simulink model "i_128w_2k_10_r310"  (Simulink 7.0)
settings: Solver=ode45  StartTime=0.0  StopTime=100000  RelTol=1e-3
undefined symbols (not defined in the file or in its folder): iBOB
libraries: xbsIndex_r4 x626, xps_library x14, xbsReplacements_r4 x12, casper_library x6, casper_library_sources x4, simulink x1
(part 1 of 6)
settings Model: Creator=dsp  LastModifiedBy=mdexter

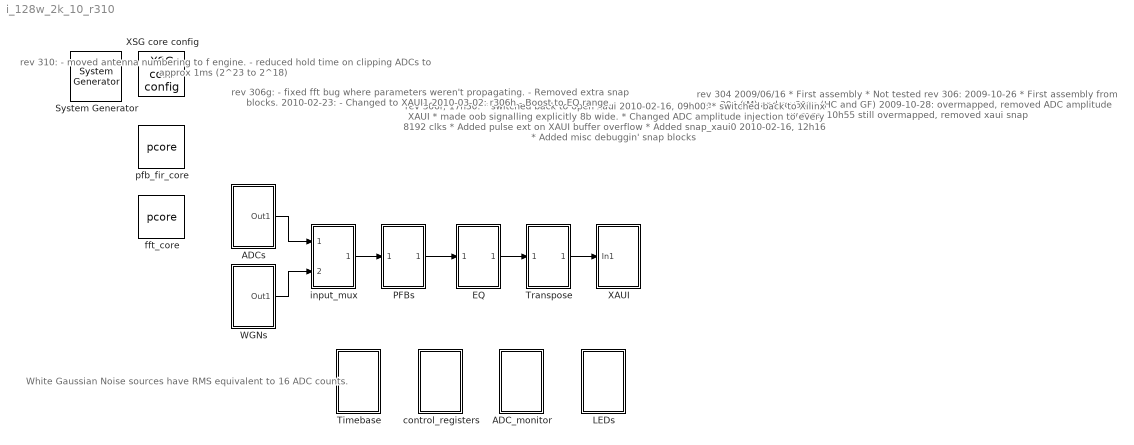
== system i_128w_2k_10_r310 ==
  note: rev 304 2009/06/16
      | * First assembly
      | * Not tested
      |
      | rev 306: 2009-10-26
      | * First assembly from rev 304 (JM) and rev305c (HC and GF)
      |
      | 2009-10-28: overmapped, removed ADC amplitude sw regs.
      | 10h55 still overmapped, removed xaui snap
  note: rev 306f, 17h30:
      |   * switched back to open xaui
      | 2010-02-16, 09h00:
      |   * switched back to Xilinx XAUI
      |   * made oob signalling explicitly 8b wide.
      |   * Changed ADC amplitude injection to every 8192 clks
      |   * Added pulse ext on XAUI buffer overflow
      |   * Added snap_xaui0
      | 2010-02-16, 12h16
      |   * Added misc debuggin' snap blocks
  note: rev 306g:
      |  - fixed fft bug where parameters
      |     weren't propagating.
      |   - Removed extra snap blocks.
      |
      | 2010-02-23:
      |   - Changed to XAUI1
      |
      | 2010-03-02: r306h
      |   - Boost to EQ range.
  note: rev 310:
      |  - moved antenna numbering to
      |    f engine.
      |  - reduced hold time on clipping
      |    ADCs to approx 1ms (2^23 to 2^18)
  note: White Gaussian Noise
      | sources have RMS
      | equivalent to 16 ADC
      | counts.
  " System Generator" : xbsIndex_r4/ System Generator  Tag=genX  SystemSampleTime=-1  xilinxfamily=virtex2p  part=xc2vp50  speed=-7  package=ff1152  synthesis_tool=XST  clock_wrapper=Clock Enables  directory=./i_128w_2k_10_r310/sysgen  testbench=off  simulink_period=1  sysclk_period=5  dcm_input_clock_period=100  incr_netlist=off  trim_vbits=Everywhere in SubSystem  dbl_ovrd=According to Block Masks  core_generation=According to Block Masks  run_coregen=off  deprecated_control=off  eval_field=0  block_type=sysgen
      settings: block_version=10.1.3
  ADC_monitor : Subsystem
  ADCs : Subsystem
  EQ : Subsystem
  LEDs : Subsystem
  PFBs : Subsystem
  Timebase : Subsystem
  Transpose : Subsystem
  WGNs : Subsystem
  XAUI : Subsystem
  XSG core config : xps_library/XSG core config  Tag=xps:xsg  SystemSampleTime=-1  hw_sys=iBOB  ibob_linux=off  clk_src=adc0_clk  iBOB_clk_src=adc0_clk  BEE2_ctrl_clk_src=sys_clk  BEE2_usr_clk_src=sys_clk  ROACH_clk_src=arb_clk  CORR_clk_src=sys_clk  gpio_clk_io_group=iBOB:sma  gpio_clk_bit_index=0  clk_rate=200  sample_period=1  synthesis_tool=XST  mpc_type=powerpc405
  control_registers : Subsystem
  fft_core : xps_library/pcore  Tag=xps:pcore  SystemSampleTime=-1  pcore_path=fft_core/fft_core.ngc
  input_mux : Subsystem
  pfb_fir_core : xps_library/pcore  Tag=xps:pcore  SystemSampleTime=-1  pcore_path=pfb_fir_core/pfb_fir_core.ngc
  wires:
  ADCs/1(Out1) -> input_mux/1(In1)
  WGNs/1(Out1) -> input_mux/2(In2)
  input_mux/1(Out1) -> PFBs/1(In1)
  PFBs/1(Out1) -> EQ/1(In1)
  EQ/1(Out1) -> Transpose/1(In1)
  Transpose/1(Out1) -> XAUI/1(In1)

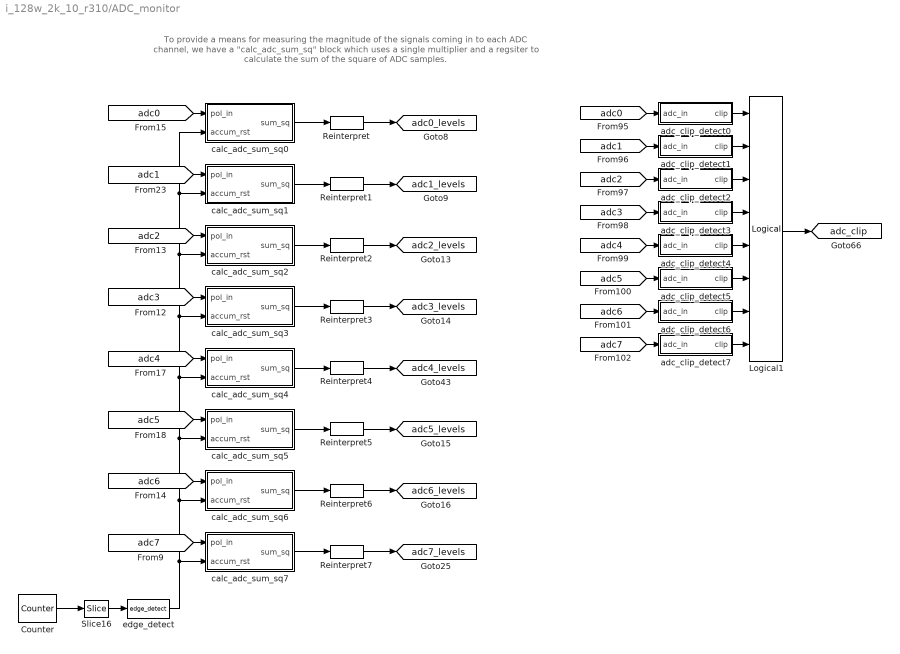
== system i_128w_2k_10_r310/ADC_monitor ==
  note: To provide a means for measuring the magnitude of the signals
      | coming in to each ADC channel, we have a "calc_adc_sum_sq"
      | block which uses a single multiplier and a regsiter to calculate
      | the sum of the square of ADC samples.
  Counter : xbsIndex_r4/Counter  cnt_type=Free Running  cnt_to=Inf  operation=Up  start_count=0  cnt_by_val=1  arith_type=Unsigned  n_bits=16  bin_pt=0  load_pin=off  rst=off  en=off  explicit_period=off  period=1  dbl_ovrd=off  use_behavioral_HDL=off  use_rpm=on  implementation=Fabric  block_type=counter
      settings: xl_area=[0, 0, 0, 0, 0, 0, 0]
  Logical1 : xbsIndex_r4/Logical  logical_function=OR  inputs=8  en=off  latency=1  precision=Full  arith_type=Unsigned  n_bits=8  bin_pt=2  align_bp=on  dbl_ovrd=off  block_type=logical
      settings: xl_area=[0, 0, 0, 0, 0, 0, 0]
  Reinterpret{,1..7} (8 alike) : xbsIndex_r4/Reinterpret  force_arith_type=on  arith_type=Unsigned  force_bin_pt=on  bin_pt=0  block_type=reinterpret
      settings: infoedit="Changes signal type without altering the binary representation.   You can changed the signal between signed and unsigned, and relocate the binary point.<P><P>Hardware notes: In hardware this block costs nothing.<P><P>Example:  Suppose the input is 6 bits wide, signed, with 2 fractional bits, and the output is forced to unsigned with 0 fractional bits.  Then an input of -2.0 (1110.00 in binary 2's complement) becomes an output of 56 (111000 in binary)."  block_version=10.1.3
  Slice16 : xbsIndex_r4/Slice  nbits=1  boolean_output=on  mode=Upper Bit Location + Width  bit1=0  base1=MSB of Input  bit0=19  base0=LSB of Input  dbl_ovrd=off  block_type=slice
      settings: infoedit="Extracts a given range of bits from each input sample and presents it at the output.  The output type is ordinarily unsigned with binary point at zero, but can be Boolean when the slice is one bit wide.<P><P>Hardware notes: In hardware this block costs nothing."  block_version=10.1.3
  adc_clip_detect0 : Subsystem  mask{n_bits=8}
      mask prompts: n_bits "Number of ADC bits"
  adc_clip_detect1 : Subsystem  mask{n_bits=8}
      mask prompts: n_bits "Number of ADC bits"
  adc_clip_detect2 : Subsystem  mask{n_bits=8}
      mask prompts: n_bits "Number of ADC bits"
  adc_clip_detect3 : Subsystem  mask{n_bits=8}
      mask prompts: n_bits "Number of ADC bits"
  adc_clip_detect4 : Subsystem  mask{n_bits=8}
      mask prompts: n_bits "Number of ADC bits"
  adc_clip_detect5 : Subsystem  mask{n_bits=8}
      mask prompts: n_bits "Number of ADC bits"
  adc_clip_detect6 : Subsystem  mask{n_bits=8}
      mask prompts: n_bits "Number of ADC bits"
  adc_clip_detect7 : Subsystem  mask{n_bits=8}
      mask prompts: n_bits "Number of ADC bits"
  calc_adc_sum_sq0 : Subsystem
  calc_adc_sum_sq1 : Subsystem
  calc_adc_sum_sq2 : Subsystem
  calc_adc_sum_sq3 : Subsystem
  calc_adc_sum_sq4 : Subsystem
  calc_adc_sum_sq5 : Subsystem
  calc_adc_sum_sq6 : Subsystem
  calc_adc_sum_sq7 : Subsystem
  edge_detect : casper_library/Misc/edge_detect  SystemSampleTime=-1  edge=Rising  polarity=Active High  x_in=[0 0.08 0.08 0.16 0.16 0.24 0.24 0.32 0.32 0.4]  y_in="[-1 -1  1  1  1  1  1  1  1  1]"  x_out=[0.6 0.68 0.68 0.76 0.76 0.84 0.84 0.92 0.92 1]  y_out="[-1 -1  1  1 -1 -1 -1 -1 -1 -1]"
      settings: AttributesFormatString=|
      | rising edges
      | active high
  tag scope: adc0_levels=global, adc1_levels=global, adc2_levels=global, adc3_levels=global, adc4_levels=global, adc5_levels=global, adc6_levels=global, adc7_levels=global, adc_clip=global
  wires:
  [adc0] -> calc_adc_sum_sq0/1(pol_in)
  calc_adc_sum_sq1/1(sum_sq) -> Reinterpret1/1
  calc_adc_sum_sq2/1(sum_sq) -> Reinterpret2/1
  calc_adc_sum_sq3/1(sum_sq) -> Reinterpret3/1
  edge_detect/1 -> calc_adc_sum_sq0/2(accum_rst), calc_adc_sum_sq1/2(accum_rst), calc_adc_sum_sq2/2(accum_rst), calc_adc_sum_sq3/2(accum_rst), calc_adc_sum_sq4/2(accum_rst), calc_adc_sum_sq5/2(accum_rst), calc_adc_sum_sq6/2(accum_rst), calc_adc_sum_sq7/2(accum_rst)
  [adc1] -> calc_adc_sum_sq1/1(pol_in)
  [adc2] -> calc_adc_sum_sq2/1(pol_in)
  [adc3] -> calc_adc_sum_sq3/1(pol_in)
  Counter/1 -> Slice16/1
  Slice16/1 -> edge_detect/1
  calc_adc_sum_sq4/1(sum_sq) -> Reinterpret4/1
  [adc4] -> calc_adc_sum_sq4/1(pol_in)
  calc_adc_sum_sq5/1(sum_sq) -> Reinterpret5/1
  calc_adc_sum_sq6/1(sum_sq) -> Reinterpret6/1
  calc_adc_sum_sq7/1(sum_sq) -> Reinterpret7/1
  [adc5] -> calc_adc_sum_sq5/1(pol_in)
  [adc6] -> calc_adc_sum_sq6/1(pol_in)
  [adc7] -> calc_adc_sum_sq7/1(pol_in)
  Reinterpret/1 -> [adc0_levels]
  Reinterpret1/1 -> [adc1_levels]
  Reinterpret2/1 -> [adc2_levels]
  Reinterpret3/1 -> [adc3_levels]
  Reinterpret4/1 -> [adc4_levels]
  Reinterpret5/1 -> [adc5_levels]
  Reinterpret6/1 -> [adc6_levels]
  Reinterpret7/1 -> [adc7_levels]
  calc_adc_sum_sq0/1(sum_sq) -> Reinterpret/1
  [adc0] -> adc_clip_detect0/1(adc_in)
  [adc1] -> adc_clip_detect1/1(adc_in)
  [adc2] -> adc_clip_detect2/1(adc_in)
  [adc3] -> adc_clip_detect3/1(adc_in)
  [adc4] -> adc_clip_detect4/1(adc_in)
  [adc5] -> adc_clip_detect5/1(adc_in)
  [adc6] -> adc_clip_detect6/1(adc_in)
  [adc7] -> adc_clip_detect7/1(adc_in)
  adc_clip_detect0/1(clip) -> Logical1/1
  adc_clip_detect1/1(clip) -> Logical1/2
  adc_clip_detect2/1(clip) -> Logical1/3
  adc_clip_detect3/1(clip) -> Logical1/4
  adc_clip_detect4/1(clip) -> Logical1/5
  adc_clip_detect5/1(clip) -> Logical1/6
  adc_clip_detect6/1(clip) -> Logical1/7
  adc_clip_detect7/1(clip) -> Logical1/8
  Logical1/1 -> [adc_clip]

== system i_128w_2k_10_r310/ADCs ==
  Band-Limited White Noise : simulink/Sources/Band-Limited White Noise  SystemSampleTime=-1  Cov=[0.1]  Ts=0.1  seed=[23341]
  Constant : Constant  Value=0
  Constant1 : Constant  OutDataType=sfix(16)  OutScaling=2^0
  Constant2 : Constant  Value=0
  Mux : Mux  Inputs=2
  Pulse Generator : DiscretePulseGenerator  Period=2^27
  Terminator11 : Terminator
  Terminator12 : Terminator
  quadc0 : xps_library/quadc  Tag=xps:quadc  SystemSampleTime=-1  adc_brd=0  adc_clk_rate=200
  quadc1 : xps_library/quadc  Tag=xps:quadc  SystemSampleTime=-1  adc_brd=1  adc_clk_rate=200
  Out1 : Outport  OutDataType=sfix(16)  OutScaling=2^0
  tag scope: adc0=global, adc1=global, adc2=global, adc3=global, adc4=global, adc5=global, adc6=global, adc7=global, sync_adc0=global, sync_adc1=global
  wires:
  quadc0/1 -> [adc0]
  quadc0/2 -> [adc1]
  quadc0/3 -> [adc2]
  quadc0/4 -> [adc3]
  quadc0/6 -> [sync_adc0]
  quadc1/1 -> [adc4]
  quadc1/2 -> [adc5]
  quadc1/3 -> [adc6]
  quadc1/4 -> [adc7]
  quadc1/6 -> [sync_adc1]
  Band-Limited White Noise/1 -> quadc1/4, quadc1/3, quadc1/2, quadc1/1, quadc0/4, quadc0/3, quadc0/2, quadc0/1
  Pulse Generator/1 -> quadc0/6, quadc1/6
  Constant1/1 -> quadc0/5, quadc1/5
  quadc0/5 -> Terminator11/1
  quadc1/5 -> Terminator12/1
  Mux/1 -> Out1/1
  Constant/1 -> Mux/1
  Constant2/1 -> Mux/2

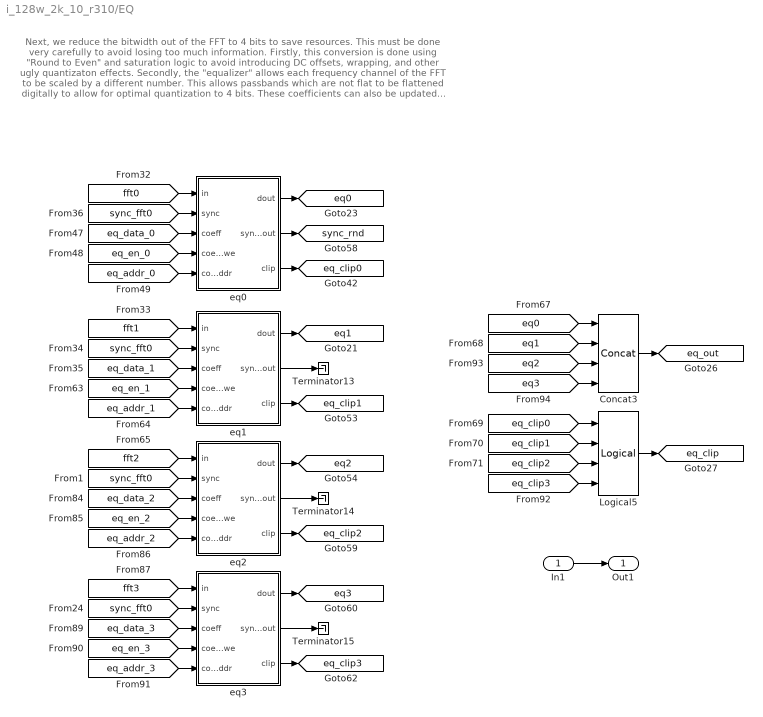
== system i_128w_2k_10_r310/EQ ==
  note: Next, we reduce the bitwidth out of the FFT to 4 bits to save resources.
      | This must be done very carefully to avoid losing too much information.
      | Firstly, this conversion is done using "Round to Even" and saturation
      | logic to avoid introducing DC offsets, wrapping, and other ugly quantizaton
      | effects.  Secondly, the "equalizer" allows each frequency channel of the
      | FFT to be scaled by a different number.  This allows passbands which are
      | not flat to be flattened digitally to allow for optimal quantization to 4 bits.
      | These coefficients can also be updated dynamically for gain control.
      | Coefficients can be dynamically written into the "equalizer" by
      | specifying the channel ("coeff_addr") and the value of the
      | coefficient ("coeff"), and then using "coeff_en" to write the
      | new coefficient into the equalization table.
  In1 : Inport  OutDataType=sfix(16)  OutScaling=2^0
  Concat3 : xbsIndex_r4/Concat  num_inputs=4  dbl_ovrd=off  block_type=concat
      settings: block_version=10.1.3
  Logical5 : xbsIndex_r4/Logical  logical_function=OR  inputs=4  en=off  latency=0  precision=Full  arith_type=Unsigned  n_bits=8  bin_pt=2  align_bp=on  dbl_ovrd=off  block_type=logical
      settings: xl_area=[0, 0, 0, 0, 0, 0, 0]
  Terminator13 : Terminator
  Terminator14 : Terminator
  Terminator15 : Terminator
  eq0 : Subsystem
  eq1 : Subsystem
  eq2 : Subsystem
  eq3 : Subsystem
  Out1 : Outport  OutDataType=sfix(16)  OutScaling=2^0
  tag scope: eq0=global, eq1=global, eq2=global, eq3=global, eq_clip0=global, eq_clip1=global, eq_clip2=global, eq_clip3=global, eq_clip=global, eq_out=global, sync_rnd=global
  wires:
  eq0/1(dout) -> [eq0]
  eq0/2(sync_out) -> [sync_rnd]
  [fft0] -> eq0/1(in)
  [eq_data_0] -> eq0/3(coeff)
  [eq_en_0] -> eq0/4(coeff_we)
  eq0/3(clip) -> [eq_clip0]
  Logical5/1 -> [eq_clip]
  Concat3/1 -> [eq_out]
  [eq_clip0] -> Logical5/1
  [eq_clip1] -> Logical5/2
  [sync_fft0] -> eq0/2(sync)
  [eq_addr_0] -> eq0/5(coeff_addr)
  [fft1] -> eq1/1(in)
  [sync_fft0] -> eq1/2(sync)
  [eq_data_1] -> eq1/3(coeff)
  [eq_en_1] -> eq1/4(coeff_we)
  [eq_addr_1] -> eq1/5(coeff_addr)
  [fft2] -> eq2/1(in)
  [sync_fft0] -> eq2/2(sync)
  [eq_data_2] -> eq2/3(coeff)
  [eq_en_2] -> eq2/4(coeff_we)
  [eq_addr_2] -> eq2/5(coeff_addr)
  [fft3] -> eq3/1(in)
  [sync_fft0] -> eq3/2(sync)
  [eq_data_3] -> eq3/3(coeff)
  [eq_en_3] -> eq3/4(coeff_we)
  [eq_addr_3] -> eq3/5(coeff_addr)
  eq1/1(dout) -> [eq1]
  eq1/2(sync_out) -> Terminator13/1
  eq1/3(clip) -> [eq_clip1]
  eq2/1(dout) -> [eq2]
  eq2/2(sync_out) -> Terminator14/1
  eq2/3(clip) -> [eq_clip2]
  eq3/1(dout) -> [eq3]
  eq3/2(sync_out) -> Terminator15/1
  eq3/3(clip) -> [eq_clip3]
  [eq_clip2] -> Logical5/3
  [eq_clip3] -> Logical5/4
  [eq0] -> Concat3/1
  [eq1] -> Concat3/2
  [eq2] -> Concat3/3
  [eq3] -> Concat3/4
  In1/1 -> Out1/1

== system i_128w_2k_10_r310/LEDs ==
  Terminator{1..5,27} (6 alike) : Terminator
  led1_arm : xps_library/gpio  Tag=xps:gpio  SystemSampleTime=-1  io_group=iBOB:led  io_dir=out  arith_type=Boolean  bitwidth=1  bin_pt=0  bit_index=1  sample_period=1  use_single_ended=off  use_ddr=off  reg_iob=on  reg_clk_phase=0  termination=None
      link override convert: arith_type=Boolean  n_bits=1  bin_pt=0
  led2_sync : xps_library/gpio  Tag=xps:gpio  SystemSampleTime=-1  io_group=iBOB:led  io_dir=out  arith_type=Boolean  bitwidth=1  bin_pt=0  bit_index=2  sample_period=1  use_single_ended=off  use_ddr=off  reg_iob=on  reg_clk_phase=0  termination=None
      link override convert: arith_type=Boolean  n_bits=1  bin_pt=0
  led4_eq_clip : xps_library/gpio  Tag=xps:gpio  SystemSampleTime=-1  io_group=iBOB:led  io_dir=out  arith_type=Boolean  bitwidth=1  bin_pt=0  bit_index=4  sample_period=1  use_single_ended=off  use_ddr=off  reg_iob=on  reg_clk_phase=0  termination=None
      link override convert: arith_type=Boolean  n_bits=1  bin_pt=0
  led5_adc_clip : xps_library/gpio  Tag=xps:gpio  SystemSampleTime=-1  io_group=iBOB:led  io_dir=out  arith_type=Boolean  bitwidth=1  bin_pt=0  bit_index=5  sample_period=1  use_single_ended=off  use_ddr=off  reg_iob=on  reg_clk_phase=0  termination=None
      link override convert: arith_type=Boolean  n_bits=1  bin_pt=0
  led6_link_dn : xps_library/gpio  Tag=xps:gpio  SystemSampleTime=-1  io_group=iBOB:led  io_dir=out  arith_type=Unsigned  bitwidth=1  bin_pt=0  bit_index=6  sample_period=1  use_single_ended=off  use_ddr=off  reg_iob=on  reg_clk_phase=0  termination=None
      link override convert: arith_type=Unsigned  n_bits=1  bin_pt=0
  led7_xaui_overlfow : xps_library/gpio  Tag=xps:gpio  SystemSampleTime=-1  io_group=iBOB:led  io_dir=out  arith_type=Unsigned  bitwidth=1  bin_pt=0  bit_index=7  sample_period=1  use_single_ended=off  use_ddr=off  reg_iob=on  reg_clk_phase=0  termination=None
      link override convert: arith_type=Unsigned  n_bits=1  bin_pt=0
  pulse_ext2 : Subsystem  mask{pulse_len=2^23}
      mask prompts: pulse_len "Length of Pulse"
      mask init:
      | bits = ceil(log2(pulse_len+1));
  pulse_ext3 : Subsystem  mask{pulse_len=2^18}
      mask prompts: pulse_len "Length of Pulse"
      mask init:
      | bits = ceil(log2(pulse_len+1));
  pulse_ext4 : Subsystem  mask{pulse_len=2^18}
      mask prompts: pulse_len "Length of Pulse"
      mask init:
      | bits = ceil(log2(pulse_len+1));
  wires:
  pulse_ext2/1(out) -> led2_sync/1
  [sync_gen] -> pulse_ext2/1(in)
  [armed] -> led1_arm/1
  [xaui_link_down] -> led6_link_dn/1
  pulse_ext4/1(out) -> led4_eq_clip/1
  [eq_clip] -> pulse_ext4/1(in)
  [xaui_buffer_overflow] -> led7_xaui_overlfow/1
  led1_arm/1 -> Terminator27/1
  led4_eq_clip/1 -> Terminator2/1
  led2_sync/1 -> Terminator3/1
  led6_link_dn/1 -> Terminator4/1
  led7_xaui_overlfow/1 -> Terminator5/1
  [adc_clip] -> pulse_ext3/1(in)
  pulse_ext3/1(out) -> led5_adc_clip/1
  led5_adc_clip/1 -> Terminator1/1

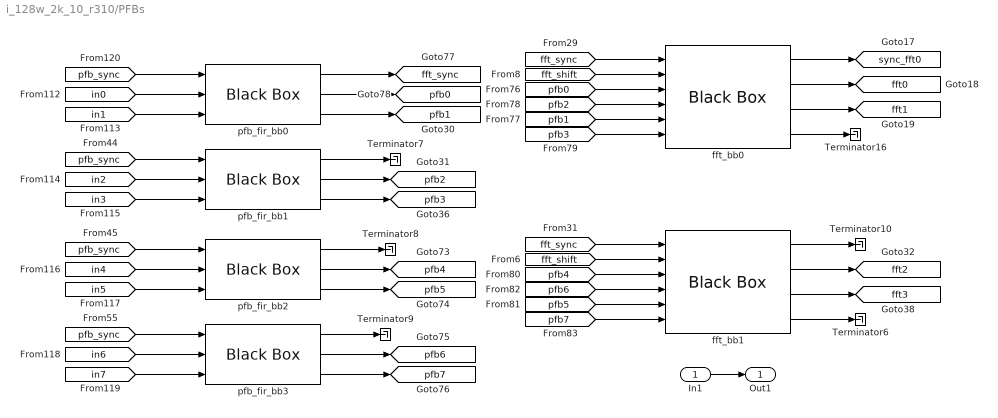
== system i_128w_2k_10_r310/PFBs ==
  In1 : Inport  OutDataType=sfix(16)  OutScaling=2^0
  Terminator{6..10,16} (6 alike) : Terminator
  fft_bb0 : xbsIndex_r4/Black Box  init_code=fft_core_config  sim_method=Inactive  block_type=blackbox2
      settings: infoedit="Incorporates black box HDL and simulation model into a System Generator design.<P><P>You must supply a Black Box with certain information about the HDL component you would like to bring into System Generator. This information is provided through a Matlab function.<P><P>When \"Simulation mode\" is set to \"Inactive\", you will typically want to provide a separate simulation model by using a Simulation Multiplexer.<P>When \"Simulation mode\" is set to \"External co-simulator\", you must include a ModelSim block in the design."  block_version=10.1.3
  fft_bb1 : xbsIndex_r4/Black Box  init_code=fft_core_config  sim_method=Inactive  block_type=blackbox2
      settings: infoedit="Incorporates black box HDL and simulation model into a System Generator design.<P><P>You must supply a Black Box with certain information about the HDL component you would like to bring into System Generator. This information is provided through a Matlab function.<P><P>When \"Simulation mode\" is set to \"Inactive\", you will typically want to provide a separate simulation model by using a Simulation Multiplexer.<P>When \"Simulation mode\" is set to \"External co-simulator\", you must include a ModelSim block in the design."  block_version=10.1.3
  pfb_fir_bb{0..3} (4 alike) : xbsIndex_r4/Black Box  init_code=pfb_fir_core_config  sim_method=Inactive  block_type=blackbox2
      settings: infoedit="Incorporates black box HDL and simulation model into a System Generator design.<P><P>You must supply a Black Box with certain information about the HDL component you would like to bring into System Generator. This information is provided through a Matlab function.<P><P>When \"Simulation mode\" is set to \"Inactive\", you will typically want to provide a separate simulation model by using a Simulation Multiplexer.<P>When \"Simulation mode\" is set to \"External co-simulator\", you must include a ModelSim block in the design."  block_version=10.1.3
  Out1 : Outport  OutDataType=sfix(16)  OutScaling=2^0
  tag scope: fft0=global, fft1=global, fft2=global, fft3=global, fft_sync=global, pfb0=global, pfb1=global, pfb2=global, pfb3=global, pfb4=global, pfb5=global, pfb6=global, pfb7=global, sync_fft0=global
  wires:
  [in0] -> pfb_fir_bb0/2
  [in1] -> pfb_fir_bb0/3
  pfb_fir_bb0/2 -> [pfb0]
  pfb_fir_bb0/3 -> [pfb1]
  [in2] -> pfb_fir_bb1/2
  [in3] -> pfb_fir_bb1/3
  [in4] -> pfb_fir_bb2/2
  [in5] -> pfb_fir_bb2/3
  [in6] -> pfb_fir_bb3/2
  [in7] -> pfb_fir_bb3/3
  pfb_fir_bb1/2 -> [pfb2]
  pfb_fir_bb1/3 -> [pfb3]
  pfb_fir_bb2/2 -> [pfb4]
  pfb_fir_bb2/3 -> [pfb5]
  pfb_fir_bb3/2 -> [pfb6]
  pfb_fir_bb3/3 -> [pfb7]
  [fft_sync] -> fft_bb1/1
  [fft_shift] -> fft_bb1/2
  fft_bb1/3 -> [fft3]
  fft_bb1/4 -> Terminator6/1
  fft_bb1/2 -> [fft2]
  fft_bb0/2 -> [fft0]
  fft_bb0/3 -> [fft1]
  fft_bb0/4 -> Terminator16/1
  fft_bb0/1 -> [sync_fft0]
  fft_bb1/1 -> Terminator10/1
  [pfb0] -> fft_bb0/3
  [pfb2] -> fft_bb0/4
  [pfb1] -> fft_bb0/5
  [pfb3] -> fft_bb0/6
  [fft_sync] -> fft_bb0/1
  [fft_shift] -> fft_bb0/2
  [pfb4] -> fft_bb1/3
  [pfb6] -> fft_bb1/4
  [pfb5] -> fft_bb1/5
  [pfb7] -> fft_bb1/6
  [pfb_sync] -> pfb_fir_bb0/1
  pfb_fir_bb0/1 -> [fft_sync]
  [pfb_sync] -> pfb_fir_bb1/1
  [pfb_sync] -> pfb_fir_bb2/1
  [pfb_sync] -> pfb_fir_bb3/1
  pfb_fir_bb1/1 -> Terminator7/1
  pfb_fir_bb2/1 -> Terminator8/1
  pfb_fir_bb3/1 -> Terminator9/1
  In1/1 -> Out1/1

== system i_128w_2k_10_r310/Timebase ==
  note: This circuit implements a scheme for synchronizing
      | multiple IBOBs to within a 200 MHz clock.  "arm_rst"
      | comes from the "ctrl" register, and indicates that the
      | next "sync_rst" should reset the sync pulse generated
      | in "sync_gen".  "sync_rst" may be generated from
      | the "ctrl" register, but more often, a 1PPS signal is
      | supplied to the "sync" input of an ADC for this
      | purpose.  Once a reset occurs, "sync_gen" generates
      | a single pulse every 2^27 clocks.  LEDs provide visual
      | confirmation that an arm and reset occur, and "mrst"
      | is passed over XAUI for the purpose of informing
      | downstream logic in a packetized correlator that
      | a "master reset" has occurred.
  Logical7 : xbsIndex_r4/Logical  logical_function=OR  inputs=3  en=off  latency=1  precision=Full  arith_type=Unsigned  n_bits=8  bin_pt=2  align_bp=on  dbl_ovrd=off  block_type=logical
      settings: xl_area=[0, 0, 0, 0, 0, 0, 0]
  sync_gen : Subsystem
  tag scope: armed=global, mrst=global, sync_gen=global
  wires:
  sync_gen/1(sync) -> [sync_gen]
  sync_gen/2(mrst) -> [mrst]
  [arm_rst] -> sync_gen/2(arm)
  [sync_rst] -> Logical7/2
  sync_gen/3(armed) -> [armed]
  Logical7/1 -> sync_gen/1(rst)
  [sync_adc0] -> Logical7/1
  [sync_adc1] -> Logical7/3

== system i_128w_2k_10_r310/Transpose ==
  note: A matrix transpose is performed in SRAM so that 128 samples of frequency
      | channel 0 are output, followed by 128 samples of channel 1, and so forth.
      | These blocks of samples for a single channel are turned into 10 GbE packets
      | on the X engine, and are then routed through a swittch.  "one_ant_a_time"
      | outputs 128 samples for channel 0 (both polarizations) of one antenna,
      | and then 128 samples for channel 0 of the other antenna, followed by
      | channel 1 of the first antenna, and so on.  This allows the X engine design to
      | pass data directly from the XAUI into a packet containing 128 time samples
      | for 1 frequency from 1 antenna.
  note: Currently "dbuf_ct_sram" double-buffers data (meaning it writes data
      | into one buffer, while reading data out in the desired order from another
      | buffer.  The number of channels in this design (2048) is limited by the
      | memory available in SRAM.  If this block were modified to be a
      | single-buffer design (see documentation for the "reorder" block for
      | ideas on how this might be done), the number of channels could
      | be doubled to 4096.
  In1 : Inport  OutDataType=sfix(16)  OutScaling=2^0
  dbuf_ct_sram : Subsystem  mask{length=11, numSpecs=7}
      mask prompts: length "Length of Spectrums (2^?) (FFT_real_2x vector length)"; numSpecs "Number of Spectrums (2^?) (pkt size in 16bit complex dual-pol words)"
      mask help: Sram transpose using double buffering method, maximum size is 256 spectrums by 2048 channels!!
  fft2x_tvg : Subsystem  mask{length=11}
      mask prompts: length "FFT_real_2x vector length (2^?)"
  one_ant_a_time : Subsystem
  sram_tvg : Subsystem
  Out1 : Outport  OutDataType=sfix(16)  OutScaling=2^0
  tag scope: ant12_pol12_reorder=global, sync_reorder=global
  wires:
  fft2x_tvg/1(dout) -> dbuf_ct_sram/1(din)
  fft2x_tvg/2(sync_out) -> dbuf_ct_sram/2(sync_in)
  sram_tvg/1(dout) -> one_ant_a_time/1(din)
  sram_tvg/2(sync_out) -> one_ant_a_time/2(sync)
  dbuf_ct_sram/1(out) -> sram_tvg/1(din)
  dbuf_ct_sram/2(sync_out) -> sram_tvg/2(sync)
  [use_sram_tvg] -> sram_tvg/3(use_tvg)
  one_ant_a_time/1(dout) -> [ant12_pol12_reorder]
  one_ant_a_time/2(sync_out) -> [sync_reorder]
  [use_fft_tvg] -> fft2x_tvg/3(use_tvg)
  [eq_out] -> fft2x_tvg/2(din)
  [sync_rnd] -> fft2x_tvg/1(sync)
  In1/1 -> Out1/1

== system i_128w_2k_10_r310/WGNs ==
  Constant : Constant  Value=0
  Constant2 : Constant  Value=0
  Mux : Mux  Inputs=2
  noise0 : Subsystem
  noise1 : Subsystem
  noise2 : Subsystem
  noise3 : Subsystem
  Out1 : Outport  OutDataType=sfix(16)  OutScaling=2^0
  tag scope: n00=global, n01=global, n10=global, n11=global, n20=global, n21=global, n30=global, n31=global
  wires:
  noise0/1(n1) -> [n00]
  noise0/2(n2) -> [n01]
  noise1/1(n1) -> [n10]
  noise1/2(n2) -> [n11]
  noise2/1(n1) -> [n20]
  noise2/2(n2) -> [n21]
  noise3/1(n1) -> [n30]
  noise3/2(n2) -> [n31]
  [seed0] -> noise0/1(seed)
  [seed3] -> noise3/1(seed)
  [seed2] -> noise2/1(seed)
  [seed1] -> noise1/1(seed)
  [seed_ld] -> noise0/2(ld)
  [seed_ld] -> noise3/2(ld)
  [seed_ld] -> noise2/2(ld)
  [seed_ld] -> noise1/2(ld)
  Mux/1 -> Out1/1
  Constant/1 -> Mux/1
  Constant2/1 -> Mux/2

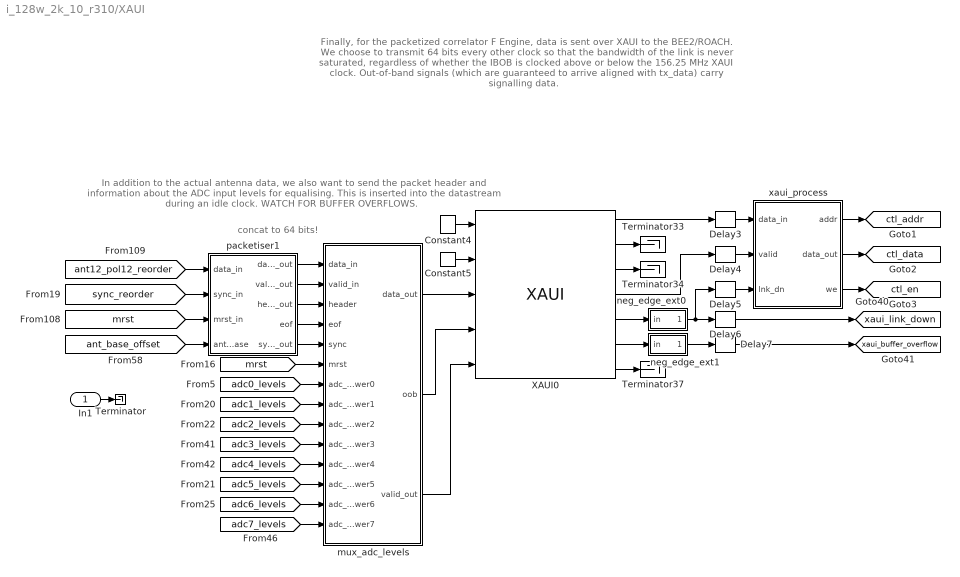
== system i_128w_2k_10_r310/XAUI ==
  note: Finally, for the packetized correlator F Engine, data is sent over
      | XAUI to the BEE2/ROACH.  We choose to transmit 64 bits every other clock
      | so that the bandwidth of the link is never saturated, regardless of whether
      | the IBOB is clocked above or below the 156.25 MHz XAUI clock.
      | Out-of-band signals (which are guaranteed to arrive aligned with
      | tx_data) carry signalling data.
  note: In addition to the actual antenna data,
      | we also want to send the packet header
      | and information about the ADC input levels for equalising.
      | This is inserted into the datastream during an idle clock.
      | WATCH FOR BUFFER OVERFLOWS.
  note: concat to 64 bits!
  In1 : Inport  OutDataType=sfix(16)  OutScaling=2^0
  Constant4 : xbsIndex_r4/Constant  arith_type=Unsigned  const=1  n_bits=1  bin_pt=0  explicit_period=on  period=1  equ=P=C  opselect=C  inp2=PCIN>>17  opr=+  inp1=P  carry=CIN  dbl_ovrd=off  block_type=constant
  Constant5 : xbsIndex_r4/Constant  arith_type=Unsigned  const=0  n_bits=1  bin_pt=0  explicit_period=on  period=1  equ=P=C  opselect=C  inp2=PCIN>>17  opr=+  inp1=P  carry=CIN  dbl_ovrd=off  block_type=constant
  Delay{3..7} (5 alike) : xbsIndex_r4/Delay  en=off  latency=1  dbl_ovrd=off  reg_retiming=on  block_type=delay
      settings: xl_area=[0, 0, 0, 0, 0, 0, 0]
  Terminator{,33..34,37} (4 alike) : Terminator
  XAUI0 : xps_library/XAUI  Tag=xps:xaui  SystemSampleTime=-1  demux=1  port=iBOB:1  open_phy=off  show_param=off  pre_emph=3  swing=800
      link override convert_tx_data: n_bits=64
      link override convert_tx_outofband: n_bits=8
      link override i_128w_2k_10_r304_XAUI0_rx_data: n_bits=64
      link override i_128w_2k_10_r304_XAUI0_rx_outofband: n_bits=8
      link override i_128w_2k_10_r306_XAUI0_rx_data: n_bits=64
      link override i_128w_2k_10_r306_XAUI0_rx_outofband: n_bits=8
      link override i_128w_2k_10_r306e_XAUI0_rx_data: n_bits=64
      link override i_128w_2k_10_r306e_XAUI0_rx_outofband: n_bits=8
      link override i_128w_2k_10_r306f_XAUI0_rx_data: n_bits=64
      link override i_128w_2k_10_r306f_XAUI0_rx_outofband: n_bits=8
      link override i_128w_2k_10_r310_XAUI0_rx_data: n_bits=64
      link override i_128w_2k_10_r310_XAUI0_rx_outofband: n_bits=8
      link override i_128w_2k_10_r310_XAUI_XAUI0_rx_data: n_bits=64
      link override i_128w_2k_10_r310_XAUI_XAUI0_rx_outofband: n_bits=8
      link override i_128w_4k_10_150_r305a_XAUI0_rx_data: n_bits=64
      link override i_128w_4k_10_150_r305a_XAUI0_rx_outofband: n_bits=8
      link override i_128w_4k_10_150_r305b_XAUI0_rx_data: n_bits=64
      link override i_128w_4k_10_150_r305b_XAUI0_rx_outofband: n_bits=8
      link override i_128w_4k_10_200_r304_XAUI0_rx_data: n_bits=64
      link override i_128w_4k_10_200_r304_XAUI0_rx_outofband: n_bits=8
      link override i_128w_4k_10_200_r305a_XAUI0_rx_data: n_bits=64
      link override i_128w_4k_10_200_r305a_XAUI0_rx_outofband: n_bits=8
      link override temp_feng_XAUI0_rx_data: n_bits=64
      link override temp_feng_XAUI0_rx_outofband: n_bits=8
  mux_adc_levels : Subsystem
  neg_edge_ext0 : Subsystem  mask{pulse_len=2^27}
      mask prompts: pulse_len "Length of Pulse"
      mask init:
      | bits = ceil(log2(pulse_len+1));
  neg_edge_ext1 : Subsystem  mask{pulse_len=2^23}
      mask prompts: pulse_len "Length of Pulse"
      mask init:
      | bits = ceil(log2(pulse_len+1));
  packetiser1 : Subsystem  mask{nwrd_bits=5, ant_bits=2}
      mask prompts: nwrd_bits "Payload length: (in 64bit words) (2^n)"; ant_bits "Number of antennas on this link (2^n)"
      mask help: Package 32 bit data into 64 bits and identify data as coming from antenna 0 or 1
  xaui_process : Subsystem
  tag scope: ctl_addr=global, ctl_data=global, ctl_en=global, xaui_buffer_overflow=global, xaui_link_down=global
  wires:
  xaui_process/2(data_out) -> [ctl_data]
  xaui_process/1(addr) -> [ctl_addr]
  Constant4/1 -> XAUI0/1
  Constant5/1 -> XAUI0/2
  XAUI0/5 -> neg_edge_ext0/1(in)
  XAUI0/4 -> Delay4/1
  neg_edge_ext0/1(out) -> Delay5/1, Delay6/1
  xaui_process/3(we) -> [ctl_en]
  XAUI0/6 -> neg_edge_ext1/1(in)
  [sync_reorder] -> packetiser1/2(sync_in)
  [mrst] -> packetiser1/3(mrst_in)
  packetiser1/1(data_out) -> mux_adc_levels/1(data_in)
  packetiser1/2(valid_out) -> mux_adc_levels/2(valid_in)
  packetiser1/3(header_out) -> mux_adc_levels/3(header)
  packetiser1/4(eof) -> mux_adc_levels/4(eof)
  packetiser1/5(sync_out) -> mux_adc_levels/5(sync)
  mux_adc_levels/1(data_out) -> XAUI0/3
  mux_adc_levels/2(oob) -> XAUI0/4
  mux_adc_levels/3(valid_out) -> XAUI0/5
  [mrst] -> mux_adc_levels/6(mrst)
  [adc0_levels] -> mux_adc_levels/7(adc_power0)
  [ant12_pol12_reorder] -> packetiser1/1(data_in)
  XAUI0/1 -> Delay3/1
  XAUI0/2 -> Terminator33/1
  XAUI0/3 -> Terminator34/1
  XAUI0/7 -> Terminator37/1
  [adc1_levels] -> mux_adc_levels/8(adc_power1)
  [adc2_levels] -> mux_adc_levels/9(adc_power2)
  [adc3_levels] -> mux_adc_levels/10(adc_power3)
  [adc4_levels] -> mux_adc_levels/11(adc_power4)
  [adc5_levels] -> mux_adc_levels/12(adc_power5)
  [adc6_levels] -> mux_adc_levels/13(adc_power6)
  [adc7_levels] -> mux_adc_levels/14(adc_power7)
  neg_edge_ext1/1(out) -> Delay7/1
  [ant_base_offset] -> packetiser1/4(ant_base)
  Delay3/1 -> xaui_process/1(data_in)
  Delay4/1 -> xaui_process/2(valid)
  Delay5/1 -> xaui_process/3(lnk_dn)
  Delay6/1 -> [xaui_link_down]
  Delay7/1 -> [xaui_buffer_overflow]
  In1/1 -> Terminator/1

== system i_128w_2k_10_r310/control_registers ==
  ctl_regs : Subsystem
  delay : Subsystem  mask{addr_offset=8195}
      mask prompts: addr_offset "Address"
      mask init:
      | start_addr = (addr_offset);
      | fmtstr = sprintf('Addr %d\n0x%04X', start_addr, start_addr);
      | set_param(gcb, 'AttributesFormatString', fmtstr);
      settings: AttributesFormatString=|
      | Addr 8195
      | 0x2003
  eq_coefs : Subsystem
  insel : Subsystem  mask{addr_offset=8194}
      mask prompts: addr_offset "Address"
      mask init:
      | start_addr = (addr_offset);
      | fmtstr = sprintf('Addr %d\n0x%04X', start_addr, start_addr);
      | set_param(gcb, 'AttributesFormatString', fmtstr);
      settings: AttributesFormatString=|
      | Addr 8194
      | 0x2002
  seed : Subsystem  mask{addr_offset=8196}
      mask prompts: addr_offset "Address"
      mask init:
      | start_addr = (addr_offset);
      | fmtstr = sprintf('Addr %d\n0x%04X', start_addr, start_addr);
      | set_param(gcb, 'AttributesFormatString', fmtstr);
      settings: AttributesFormatString=|
      | Addr 8196
      | 0x2004

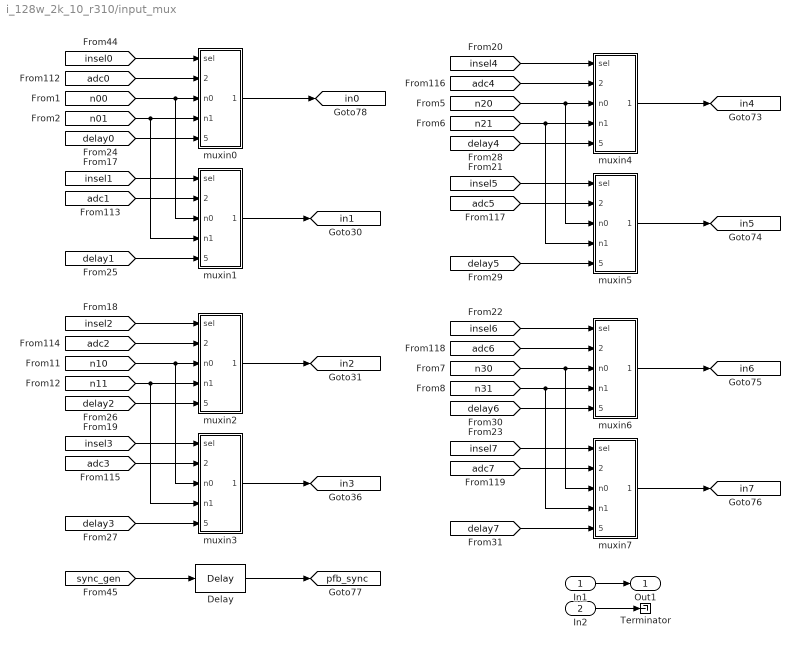
== system i_128w_2k_10_r310/input_mux ==
  In1 : Inport  OutDataType=sfix(16)  OutScaling=2^0
  In2 : Inport  Port=2  OutDataType=sfix(16)  OutScaling=2^0
  Delay : xbsIndex_r4/Delay  en=off  latency=2  dbl_ovrd=off  reg_retiming=off  block_type=delay
  Terminator : Terminator
  muxin0 : Subsystem
  muxin1 : Subsystem
  muxin2 : Subsystem
  muxin3 : Subsystem
  muxin4 : Subsystem
  muxin5 : Subsystem
  muxin6 : Subsystem
  muxin7 : Subsystem
  Out1 : Outport  OutDataType=sfix(16)  OutScaling=2^0
  tag scope: in0=global, in1=global, in2=global, in3=global, in4=global, in5=global, in6=global, in7=global, pfb_sync=global
  wires:
  [insel0] -> muxin0/1(sel)
  [adc0] -> muxin0/2(adc)
  [n00] -> muxin0/3(n0), muxin1/3(n0)
  [n01] -> muxin0/4(n1), muxin1/4(n1)
  [delay0] -> muxin0/5(delay)
  muxin0/1(out) -> [in0]
  [insel1] -> muxin1/1(sel)
  [adc1] -> muxin1/2(adc)
  [delay1] -> muxin1/5(delay)
  [insel2] -> muxin2/1(sel)
  [adc2] -> muxin2/2(adc)
  [n10] -> muxin3/3(n0), muxin2/3(n0)
  [n11] -> muxin3/4(n1), muxin2/4(n1)
  [delay2] -> muxin2/5(delay)
  [insel3] -> muxin3/1(sel)
  [adc3] -> muxin3/2(adc)
  [delay3] -> muxin3/5(delay)
  muxin1/1(out) -> [in1]
  muxin2/1(out) -> [in2]
  muxin3/1(out) -> [in3]
  [insel4] -> muxin4/1(sel)
  [adc4] -> muxin4/2(adc)
  [n20] -> muxin5/3(n0), muxin4/3(n0)
  [n21] -> muxin5/4(n1), muxin4/4(n1)
  [delay4] -> muxin4/5(delay)
  [insel5] -> muxin5/1(sel)
  [adc5] -> muxin5/2(adc)
  [delay5] -> muxin5/5(delay)
  [insel6] -> muxin6/1(sel)
  [adc6] -> muxin6/2(adc)
  [n30] -> muxin7/3(n0), muxin6/3(n0)
  [n31] -> muxin7/4(n1), muxin6/4(n1)
  [delay6] -> muxin6/5(delay)
  [insel7] -> muxin7/1(sel)
  [adc7] -> muxin7/2(adc)
  [delay7] -> muxin7/5(delay)
  muxin7/1(out) -> [in7]
  muxin4/1(out) -> [in4]
  muxin5/1(out) -> [in5]
  muxin6/1(out) -> [in6]
  [sync_gen] -> Delay/1
  Delay/1 -> [pfb_sync]
  In1/1 -> Out1/1
  In2/1 -> Terminator/1

== system i_128w_2k_10_r310/ADC_monitor/adc_clip_detect0 ==
  adc_in : Inport
  Constant : xbsIndex_r4/Constant  arith_type=Unsigned  const=((2^(n_bits-1)-1)/(2^(n_bits-1)))^2  n_bits=2*n_bits +1  bin_pt=n_bits*2  explicit_period=on  period=1  equ=P=C  opselect=C  inp2=PCIN>>17  opr=+  inp1=P  carry=CIN  dbl_ovrd=off  block_type=constant
  Mult : xbsIndex_r4/Mult  precision=Full  arith_type="Signed  (2's comp)"  n_bits=16  bin_pt=14  quantization=Truncate  overflow=Wrap  en=off  latency=3  dbl_ovrd=off  use_behavioral_HDL=off  use_embedded=on  opt=Speed  optimum_pipeline=on  pipeline=on  use_rpm=on  placement_style=Triangular  block_type=mult
      settings: infoedit=Hardware notes: To use the internal pipeline stage of the dedicated multiplier you must select 'Pipeline for maximum performance'.  block_version=10.1.3
  Relational : xbsIndex_r4/Relational  mode=a>=b  en=off  latency=1  dbl_ovrd=off  block_type=relational
      settings: block_version=10.1.3
  clip : Outport
  wires:
  adc_in/1 -> Mult/2, Mult/1
  Mult/1 -> Relational/1
  Constant/1 -> Relational/2
  Relational/1 -> clip/1

== system i_128w_2k_10_r310/ADC_monitor/adc_clip_detect1 ==
  adc_in : Inport
  Constant : xbsIndex_r4/Constant  arith_type=Unsigned  const=((2^(n_bits-1)-1)/(2^(n_bits-1)))^2  n_bits=2*n_bits +1  bin_pt=n_bits*2  explicit_period=on  period=1  equ=P=C  opselect=C  inp2=PCIN>>17  opr=+  inp1=P  carry=CIN  dbl_ovrd=off  block_type=constant
  Mult : xbsIndex_r4/Mult  precision=Full  arith_type="Signed  (2's comp)"  n_bits=16  bin_pt=14  quantization=Truncate  overflow=Wrap  en=off  latency=3  dbl_ovrd=off  use_behavioral_HDL=off  use_embedded=on  opt=Speed  optimum_pipeline=on  pipeline=on  use_rpm=on  placement_style=Triangular  block_type=mult
      settings: infoedit=Hardware notes: To use the internal pipeline stage of the dedicated multiplier you must select 'Pipeline for maximum performance'.  block_version=10.1.3
  Relational : xbsIndex_r4/Relational  mode=a>=b  en=off  latency=1  dbl_ovrd=off  block_type=relational
      settings: block_version=10.1.3
  clip : Outport
  wires:
  Relational/1 -> clip/1
  Constant/1 -> Relational/2
  Mult/1 -> Relational/1
  adc_in/1 -> Mult/1, Mult/2

== system i_128w_2k_10_r310/ADC_monitor/adc_clip_detect2 ==
  adc_in : Inport
  Constant : xbsIndex_r4/Constant  arith_type=Unsigned  const=((2^(n_bits-1)-1)/(2^(n_bits-1)))^2  n_bits=2*n_bits +1  bin_pt=n_bits*2  explicit_period=on  period=1  equ=P=C  opselect=C  inp2=PCIN>>17  opr=+  inp1=P  carry=CIN  dbl_ovrd=off  block_type=constant
  Mult : xbsIndex_r4/Mult  precision=Full  arith_type="Signed  (2's comp)"  n_bits=16  bin_pt=14  quantization=Truncate  overflow=Wrap  en=off  latency=3  dbl_ovrd=off  use_behavioral_HDL=off  use_embedded=on  opt=Speed  optimum_pipeline=on  pipeline=on  use_rpm=on  placement_style=Triangular  block_type=mult
      settings: infoedit=Hardware notes: To use the internal pipeline stage of the dedicated multiplier you must select 'Pipeline for maximum performance'.  block_version=10.1.3
  Relational : xbsIndex_r4/Relational  mode=a>=b  en=off  latency=1  dbl_ovrd=off  block_type=relational
      settings: block_version=10.1.3
  clip : Outport
  wires:
  adc_in/1 -> Mult/2, Mult/1
  Mult/1 -> Relational/1
  Constant/1 -> Relational/2
  Relational/1 -> clip/1

== system i_128w_2k_10_r310/ADC_monitor/adc_clip_detect3 ==
  adc_in : Inport
  Constant : xbsIndex_r4/Constant  arith_type=Unsigned  const=((2^(n_bits-1)-1)/(2^(n_bits-1)))^2  n_bits=2*n_bits +1  bin_pt=n_bits*2  explicit_period=on  period=1  equ=P=C  opselect=C  inp2=PCIN>>17  opr=+  inp1=P  carry=CIN  dbl_ovrd=off  block_type=constant
  Mult : xbsIndex_r4/Mult  precision=Full  arith_type="Signed  (2's comp)"  n_bits=16  bin_pt=14  quantization=Truncate  overflow=Wrap  en=off  latency=3  dbl_ovrd=off  use_behavioral_HDL=off  use_embedded=on  opt=Speed  optimum_pipeline=on  pipeline=on  use_rpm=on  placement_style=Triangular  block_type=mult
      settings: infoedit=Hardware notes: To use the internal pipeline stage of the dedicated multiplier you must select 'Pipeline for maximum performance'.  block_version=10.1.3
  Relational : xbsIndex_r4/Relational  mode=a>=b  en=off  latency=1  dbl_ovrd=off  block_type=relational
      settings: block_version=10.1.3
  clip : Outport
  wires:
  Relational/1 -> clip/1
  Constant/1 -> Relational/2
  Mult/1 -> Relational/1
  adc_in/1 -> Mult/1, Mult/2

== system i_128w_2k_10_r310/ADC_monitor/adc_clip_detect4 ==
  adc_in : Inport
  Constant : xbsIndex_r4/Constant  arith_type=Unsigned  const=((2^(n_bits-1)-1)/(2^(n_bits-1)))^2  n_bits=2*n_bits +1  bin_pt=n_bits*2  explicit_period=on  period=1  equ=P=C  opselect=C  inp2=PCIN>>17  opr=+  inp1=P  carry=CIN  dbl_ovrd=off  block_type=constant
  Mult : xbsIndex_r4/Mult  precision=Full  arith_type="Signed  (2's comp)"  n_bits=16  bin_pt=14  quantization=Truncate  overflow=Wrap  en=off  latency=3  dbl_ovrd=off  use_behavioral_HDL=off  use_embedded=on  opt=Speed  optimum_pipeline=on  pipeline=on  use_rpm=on  placement_style=Triangular  block_type=mult
      settings: infoedit=Hardware notes: To use the internal pipeline stage of the dedicated multiplier you must select 'Pipeline for maximum performance'.  block_version=10.1.3
  Relational : xbsIndex_r4/Relational  mode=a>=b  en=off  latency=1  dbl_ovrd=off  block_type=relational
      settings: block_version=10.1.3
  clip : Outport
  wires:
  Relational/1 -> clip/1
  Constant/1 -> Relational/2
  Mult/1 -> Relational/1
  adc_in/1 -> Mult/1, Mult/2

== system i_128w_2k_10_r310/ADC_monitor/adc_clip_detect5 ==
  adc_in : Inport
  Constant : xbsIndex_r4/Constant  arith_type=Unsigned  const=((2^(n_bits-1)-1)/(2^(n_bits-1)))^2  n_bits=2*n_bits +1  bin_pt=n_bits*2  explicit_period=on  period=1  equ=P=C  opselect=C  inp2=PCIN>>17  opr=+  inp1=P  carry=CIN  dbl_ovrd=off  block_type=constant
  Mult : xbsIndex_r4/Mult  precision=Full  arith_type="Signed  (2's comp)"  n_bits=16  bin_pt=14  quantization=Truncate  overflow=Wrap  en=off  latency=3  dbl_ovrd=off  use_behavioral_HDL=off  use_embedded=on  opt=Speed  optimum_pipeline=on  pipeline=on  use_rpm=on  placement_style=Triangular  block_type=mult
      settings: infoedit=Hardware notes: To use the internal pipeline stage of the dedicated multiplier you must select 'Pipeline for maximum performance'.  block_version=10.1.3
  Relational : xbsIndex_r4/Relational  mode=a>=b  en=off  latency=1  dbl_ovrd=off  block_type=relational
      settings: block_version=10.1.3
  clip : Outport
  wires:
  adc_in/1 -> Mult/2, Mult/1
  Mult/1 -> Relational/1
  Constant/1 -> Relational/2
  Relational/1 -> clip/1

== system i_128w_2k_10_r310/ADC_monitor/adc_clip_detect6 ==
  adc_in : Inport
  Constant : xbsIndex_r4/Constant  arith_type=Unsigned  const=((2^(n_bits-1)-1)/(2^(n_bits-1)))^2  n_bits=2*n_bits +1  bin_pt=n_bits*2  explicit_period=on  period=1  equ=P=C  opselect=C  inp2=PCIN>>17  opr=+  inp1=P  carry=CIN  dbl_ovrd=off  block_type=constant
  Mult : xbsIndex_r4/Mult  precision=Full  arith_type="Signed  (2's comp)"  n_bits=16  bin_pt=14  quantization=Truncate  overflow=Wrap  en=off  latency=3  dbl_ovrd=off  use_behavioral_HDL=off  use_embedded=on  opt=Speed  optimum_pipeline=on  pipeline=on  use_rpm=on  placement_style=Triangular  block_type=mult
      settings: infoedit=Hardware notes: To use the internal pipeline stage of the dedicated multiplier you must select 'Pipeline for maximum performance'.  block_version=10.1.3
  Relational : xbsIndex_r4/Relational  mode=a>=b  en=off  latency=1  dbl_ovrd=off  block_type=relational
      settings: block_version=10.1.3
  clip : Outport
  wires:
  Relational/1 -> clip/1
  Constant/1 -> Relational/2
  Mult/1 -> Relational/1
  adc_in/1 -> Mult/1, Mult/2

== system i_128w_2k_10_r310/ADC_monitor/adc_clip_detect7 ==
  adc_in : Inport
  Constant : xbsIndex_r4/Constant  arith_type=Unsigned  const=((2^(n_bits-1)-1)/(2^(n_bits-1)))^2  n_bits=2*n_bits +1  bin_pt=n_bits*2  explicit_period=on  period=1  equ=P=C  opselect=C  inp2=PCIN>>17  opr=+  inp1=P  carry=CIN  dbl_ovrd=off  block_type=constant
  Mult : xbsIndex_r4/Mult  precision=Full  arith_type="Signed  (2's comp)"  n_bits=16  bin_pt=14  quantization=Truncate  overflow=Wrap  en=off  latency=3  dbl_ovrd=off  use_behavioral_HDL=off  use_embedded=on  opt=Speed  optimum_pipeline=on  pipeline=on  use_rpm=on  placement_style=Triangular  block_type=mult
      settings: infoedit=Hardware notes: To use the internal pipeline stage of the dedicated multiplier you must select 'Pipeline for maximum performance'.  block_version=10.1.3
  Relational : xbsIndex_r4/Relational  mode=a>=b  en=off  latency=1  dbl_ovrd=off  block_type=relational
      settings: block_version=10.1.3
  clip : Outport
  wires:
  adc_in/1 -> Mult/2, Mult/1
  Mult/1 -> Relational/1
  Constant/1 -> Relational/2
  Relational/1 -> clip/1

== system i_128w_2k_10_r310/ADC_monitor/calc_adc_sum_sq0 ==
  pol_in : Inport  OutDataType=sfix(16)  OutScaling=2^0
  accum_rst : Inport  Port=2  OutDataType=sfix(16)  OutScaling=2^0
  Accumulator : xbsIndex_r4/Accumulator  operation=Add  n_bits=32  overflow=Wrap  scale=1  rst=on  hasbypass=off  en=off  dbl_ovrd=off  use_behavioral_HDL=on  implementation=Fabric  block_type=accum
      settings: infoedit="Adder or subtractor-based accumulator.   Output type and binary point position match the input.<P><P>Hardware notes: When \"Reinitialize with input 'b' on reset\" is selected, the accumulator is forced to run at the system rate even if the input 'b' is running at a slower rate."  xl_area=[0, 0, 0, 0, 0, 0, 0]  block_version=10.1.3
  Mult : xbsIndex_r4/Mult  precision=Full  arith_type="Signed  (2's comp)"  n_bits=8  bin_pt=2  quantization=Truncate  overflow=Wrap  en=off  latency=2  dbl_ovrd=off  use_behavioral_HDL=on  use_embedded=on  opt=Speed  optimum_pipeline=on  pipeline=on  use_rpm=on  placement_style=Rectangular shape  block_type=mult
      settings: infoedit=Hardware notes: To use the internal pipeline stage of the dedicated multiplier you must select 'Pipeline for maximum performance'.  xl_area=[0, 0, 0, 0, 0, 0, 0]  block_version=10.1.3
  Register : xbsIndex_r4/Register  init=0  rst=off  en=on  dbl_ovrd=off  block_type=register
      settings: xl_area=[0, 0, 0, 0, 0, 0, 0]
  sum_sq : Outport  OutDataType=sfix(16)  OutScaling=2^0
  wires:
  pol_in/1 -> Mult/2, Mult/1
  accum_rst/1 -> Register/2, Accumulator/2
  Register/1 -> sum_sq/1
  Accumulator/1 -> Register/1
  Mult/1 -> Accumulator/1

== system i_128w_2k_10_r310/ADC_monitor/calc_adc_sum_sq1 ==
  pol_in : Inport  OutDataType=sfix(16)  OutScaling=2^0
  accum_rst : Inport  Port=2  OutDataType=sfix(16)  OutScaling=2^0
  Accumulator : xbsIndex_r4/Accumulator  operation=Add  n_bits=32  overflow=Wrap  scale=1  rst=on  hasbypass=off  en=off  dbl_ovrd=off  use_behavioral_HDL=on  implementation=Fabric  block_type=accum
      settings: infoedit="Adder or subtractor-based accumulator.   Output type and binary point position match the input.<P><P>Hardware notes: When \"Reinitialize with input 'b' on reset\" is selected, the accumulator is forced to run at the system rate even if the input 'b' is running at a slower rate."  xl_area=[0, 0, 0, 0, 0, 0, 0]  block_version=10.1.3
  Mult : xbsIndex_r4/Mult  precision=Full  arith_type="Signed  (2's comp)"  n_bits=8  bin_pt=2  quantization=Truncate  overflow=Wrap  en=off  latency=2  dbl_ovrd=off  use_behavioral_HDL=on  use_embedded=on  opt=Speed  optimum_pipeline=on  pipeline=on  use_rpm=on  placement_style=Rectangular shape  block_type=mult
      settings: infoedit=Hardware notes: To use the internal pipeline stage of the dedicated multiplier you must select 'Pipeline for maximum performance'.  xl_area=[0, 0, 0, 0, 0, 0, 0]  block_version=10.1.3
  Register : xbsIndex_r4/Register  init=0  rst=off  en=on  dbl_ovrd=off  block_type=register
      settings: xl_area=[0, 0, 0, 0, 0, 0, 0]
  sum_sq : Outport  OutDataType=sfix(16)  OutScaling=2^0
  wires:
  Mult/1 -> Accumulator/1
  Accumulator/1 -> Register/1
  Register/1 -> sum_sq/1
  accum_rst/1 -> Accumulator/2, Register/2
  pol_in/1 -> Mult/1, Mult/2

== system i_128w_2k_10_r310/ADC_monitor/calc_adc_sum_sq2 ==
  pol_in : Inport  OutDataType=sfix(16)  OutScaling=2^0
  accum_rst : Inport  Port=2  OutDataType=sfix(16)  OutScaling=2^0
  Accumulator : xbsIndex_r4/Accumulator  operation=Add  n_bits=32  overflow=Wrap  scale=1  rst=on  hasbypass=off  en=off  dbl_ovrd=off  use_behavioral_HDL=on  implementation=Fabric  block_type=accum
      settings: infoedit="Adder or subtractor-based accumulator.   Output type and binary point position match the input.<P><P>Hardware notes: When \"Reinitialize with input 'b' on reset\" is selected, the accumulator is forced to run at the system rate even if the input 'b' is running at a slower rate."  xl_area=[0, 0, 0, 0, 0, 0, 0]  block_version=10.1.3
  Mult : xbsIndex_r4/Mult  precision=Full  arith_type="Signed  (2's comp)"  n_bits=8  bin_pt=2  quantization=Truncate  overflow=Wrap  en=off  latency=2  dbl_ovrd=off  use_behavioral_HDL=on  use_embedded=on  opt=Speed  optimum_pipeline=on  pipeline=on  use_rpm=on  placement_style=Rectangular shape  block_type=mult
      settings: infoedit=Hardware notes: To use the internal pipeline stage of the dedicated multiplier you must select 'Pipeline for maximum performance'.  xl_area=[0, 0, 0, 0, 0, 0, 0]  block_version=10.1.3
  Register : xbsIndex_r4/Register  init=0  rst=off  en=on  dbl_ovrd=off  block_type=register
      settings: xl_area=[0, 0, 0, 0, 0, 0, 0]
  sum_sq : Outport  OutDataType=sfix(16)  OutScaling=2^0
  wires:
  pol_in/1 -> Mult/2, Mult/1
  accum_rst/1 -> Register/2, Accumulator/2
  Register/1 -> sum_sq/1
  Accumulator/1 -> Register/1
  Mult/1 -> Accumulator/1

== system i_128w_2k_10_r310/ADC_monitor/calc_adc_sum_sq3 ==
  pol_in : Inport  OutDataType=sfix(16)  OutScaling=2^0
  accum_rst : Inport  Port=2  OutDataType=sfix(16)  OutScaling=2^0
  Accumulator : xbsIndex_r4/Accumulator  operation=Add  n_bits=32  overflow=Wrap  scale=1  rst=on  hasbypass=off  en=off  dbl_ovrd=off  use_behavioral_HDL=on  implementation=Fabric  block_type=accum
      settings: infoedit="Adder or subtractor-based accumulator.   Output type and binary point position match the input.<P><P>Hardware notes: When \"Reinitialize with input 'b' on reset\" is selected, the accumulator is forced to run at the system rate even if the input 'b' is running at a slower rate."  xl_area=[0, 0, 0, 0, 0, 0, 0]  block_version=10.1.3
  Mult : xbsIndex_r4/Mult  precision=Full  arith_type="Signed  (2's comp)"  n_bits=8  bin_pt=2  quantization=Truncate  overflow=Wrap  en=off  latency=2  dbl_ovrd=off  use_behavioral_HDL=on  use_embedded=on  opt=Speed  optimum_pipeline=on  pipeline=on  use_rpm=on  placement_style=Rectangular shape  block_type=mult
      settings: infoedit=Hardware notes: To use the internal pipeline stage of the dedicated multiplier you must select 'Pipeline for maximum performance'.  xl_area=[0, 0, 0, 0, 0, 0, 0]  block_version=10.1.3
  Register : xbsIndex_r4/Register  init=0  rst=off  en=on  dbl_ovrd=off  block_type=register
      settings: xl_area=[0, 0, 0, 0, 0, 0, 0]
  sum_sq : Outport  OutDataType=sfix(16)  OutScaling=2^0
  wires:
  Mult/1 -> Accumulator/1
  Accumulator/1 -> Register/1
  Register/1 -> sum_sq/1
  accum_rst/1 -> Accumulator/2, Register/2
  pol_in/1 -> Mult/1, Mult/2

== system i_128w_2k_10_r310/ADC_monitor/calc_adc_sum_sq4 ==
  pol_in : Inport  OutDataType=sfix(16)  OutScaling=2^0
  accum_rst : Inport  Port=2  OutDataType=sfix(16)  OutScaling=2^0
  Accumulator : xbsIndex_r4/Accumulator  operation=Add  n_bits=32  overflow=Wrap  scale=1  rst=on  hasbypass=off  en=off  dbl_ovrd=off  use_behavioral_HDL=on  implementation=Fabric  block_type=accum
      settings: infoedit="Adder or subtractor-based accumulator.   Output type and binary point position match the input.<P><P>Hardware notes: When \"Reinitialize with input 'b' on reset\" is selected, the accumulator is forced to run at the system rate even if the input 'b' is running at a slower rate."  xl_area=[0, 0, 0, 0, 0, 0, 0]  block_version=10.1.3
  Mult : xbsIndex_r4/Mult  precision=Full  arith_type="Signed  (2's comp)"  n_bits=8  bin_pt=2  quantization=Truncate  overflow=Wrap  en=off  latency=2  dbl_ovrd=off  use_behavioral_HDL=on  use_embedded=on  opt=Speed  optimum_pipeline=on  pipeline=on  use_rpm=on  placement_style=Rectangular shape  block_type=mult
      settings: infoedit=Hardware notes: To use the internal pipeline stage of the dedicated multiplier you must select 'Pipeline for maximum performance'.  xl_area=[0, 0, 0, 0, 0, 0, 0]  block_version=10.1.3
  Register : xbsIndex_r4/Register  init=0  rst=off  en=on  dbl_ovrd=off  block_type=register
      settings: xl_area=[0, 0, 0, 0, 0, 0, 0]
  sum_sq : Outport  OutDataType=sfix(16)  OutScaling=2^0
  wires:
  pol_in/1 -> Mult/2, Mult/1
  accum_rst/1 -> Register/2, Accumulator/2
  Register/1 -> sum_sq/1
  Accumulator/1 -> Register/1
  Mult/1 -> Accumulator/1
